simulink model "Assign_Task3and4"  (R2024a)
settings: Solver=ode1  StartTime=0.0  StopTime=simTime  FixedStep=Ts  MaxStep=Ts  RelTol=1e-3
model workspace (MAT data in the model file):
  wsw = 2000
values from neighbouring files (symbols this model uses):
  fg = 50    [Parameters.m]
  generator_inertia = 5    [Parameters.m]
  kd = 0    [Parameters.m]
  ki = 0    [Parameters.m]
  kp = 1/R    (= 20)    [Parameters.m]
  R = 0.05    [Parameters.m]
  S0non = 1000e6    (= 1000000000)    [Parameters.m]
  simTime = 60    [Parameters.m]
  Ts = 20e-6    (= 2e-05)    [Parameters.m]
  Vhv = 22e3    (= 22000)    [Parameters.m]
  Vmv = 22e3    (= 22000)    [Parameters.m]
libraries: simulink_extras x8, spsCurrentMeasurementLib x6, spsGroundLib x6, spsVoltageMeasurementLib x6, spsThreePhaseParallelRLCLoadLib x6, simulink x3, spsPower3phInstantaneousLib x2, spsSynchronousMachinepuStandardLib x2, spsThreePhaseBreakerLib x2, spsThreePhaseDynamicLoadLib x1, slpidlib x1, eeGeneralControl x1
settings Model: Creator=Vinicius  LastModifiedBy=citcea
settings SolverCC: AlgebraicLoopSolver=TrustRegion
settings DataIOCC: InitialState=out_EMTsteady50VSC.xFinal  SaveOperatingPoint=on  SaveOutput=off  SignalLogging=off  DSMLogging=off  TimeSaveName=t
settings OptimizationCC: BlockReduction=off
settings ModelReferenceCC: EnableRefExpFcnMdlSchedulingChecks=on
settings RTWCC: BuildConfiguration=Faster Runs  GPUComputeCapability=3.5  DLArmComputeVersion=19.05

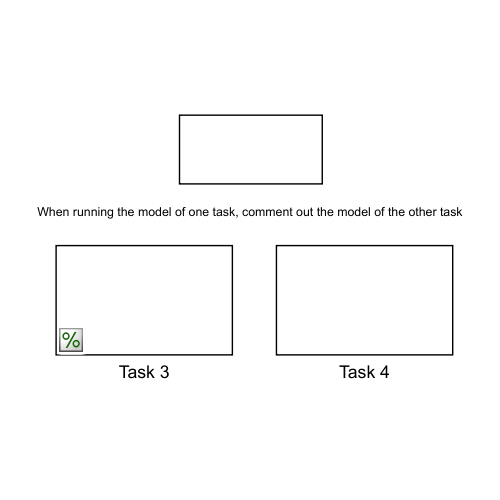
[thumbnail: Simulink's stored preview of the top-level diagram]
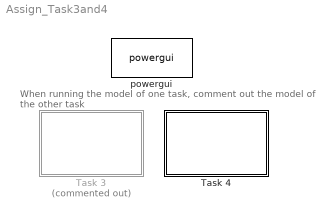
== system Assign_Task3and4 ==
  note: When running the model of one task, comment out the model of the other task
  Task 3 : Subsystem  Commented=on
  Task 4 : Subsystem
  powergui : sps_lib/powergui  Priority=1  SimulationMode=Discrete  SampleTime=Ts  frequency=60  Iterations=50  frequencyindice=50  Pbase=100e6  ErrMax=0.0001  UnitsV=kV  UnitsW=MW  buscounter=0  FunctionMessages=off  echomessages=off  EnableUseOfTLC=off  CurrentSourceSwitches=off  DisableSnubberDevices=off  DisableRonSwitches=off  DisableVfSwitches=off  DisplayEquations=off  AutomaticDiscreteSolvers=off  SolverType=Tustin/Backward Euler (TBE)  Interpol=off  ExternalGateDelay=off  methode=off  Ts=100  x0status=blocks  SPID=on  SwTol=0  HookPort=off  NonlinearTolerance=1e-4  nMaxIteration=100  ContinueOnMaxIteration=off  RestoreLinks=warning  ResistiveCurrentMeasurement=off  Frange=[0:2:500]  Ylog=off  Xlog=on  ShowGrid=off  save=off  variable=ZData  structure=0  ZoomFFT=off  StartTime=0.0  cycles=1  DisplayStyle=1  fundamental=60  FreqAxis=off  MaxFrequency=1000  frequencyindicesteady=1  RmsSteady=1  display=off

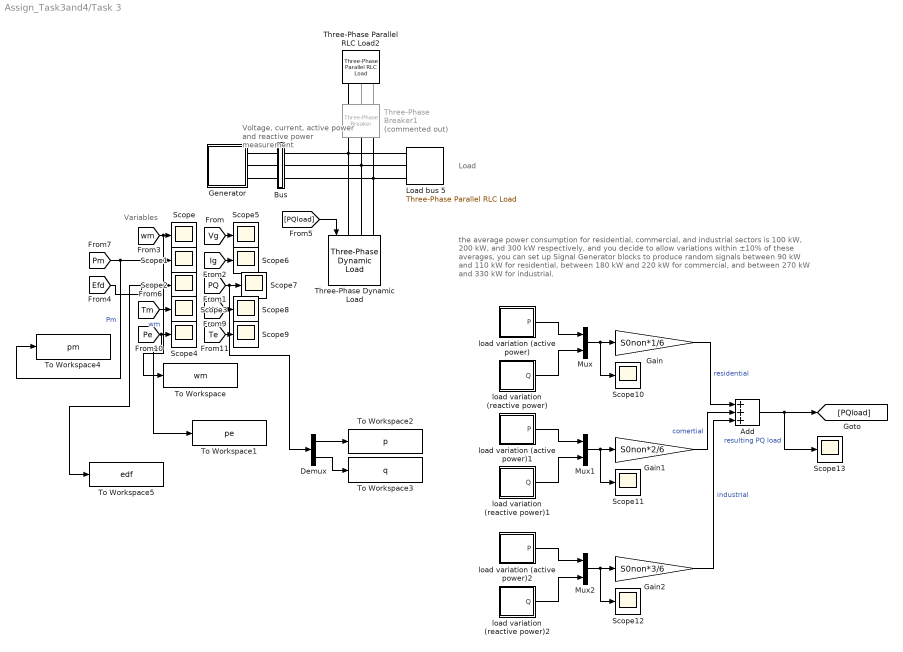
== system Assign_Task3and4/Task 3 ==
  note: the average power consumption for residential, commercial, and industrial sectors is 100 kW, 200 kW, and 300 kW respectively, and you decide to allow variations within ±10% of these averages, you can set up Signal Generator blocks to produce random signals between 90 kW and 110 kW for residential, between 180 kW and 220 kW for commercial, and between 270 kW and 330 kW for industrial.
  note: Variables
  note: Voltage, current, active power and reactive power measurement
  note: Load
  Add : Sum  Inputs=+++
  Bus : Subsystem
  Demux : Demux  Outputs=2
  Gain : Gain  Gain=S0non*1/6
  Gain1 : Gain  Gain=S0non*2/6
  Gain2 : Gain  Gain=S0non*3/6
  Generator : Subsystem
      mask Display: disp('SG')
  Load bus 5 : spsThreePhaseParallelRLCLoadLib/Three-Phase Parallel RLC Load  LConnTagsString=A|B|C  Configuration=Y (grounded)  NominalVoltage=Vmv  Vabc=[1e3 1e3 1e3]  Vabcp=[1e3 1e3 1e3]  NominalFrequency=fg  UnbalancedPower=off  ActivePower=300e6  InductivePower=50e6  CapacitivePower=0  Pabc=[10e3 9e3 11e3]  QLabc=[100 90 110]  QCabc=[100 90 110]  Pabcp=[10e3 9e3 11e3]  QLabcp=[100 90 110]  QCabcp=[100 90 110]  Measurements=None  LoadType=constant PQ
  Mux : Mux  Inputs=2
  Mux1 : Mux  Inputs=2
  Mux2 : Mux  Inputs=2
  Scope{,1..13} (14 alike) : Scope
  Three-Phase Dynamic Load : spsThreePhaseDynamicLoadLib/Three-Phase Dynamic Load  NominalVoltage=[Vmv 50 ]  ActiveReactivePowers=[0.3 0.01]*S0non  PositiveSequence=[1.0 0]  ExternalControl=on  NpNq=[1.3 2]  TimeConstants="[0  0  0  0]"  MinimumVoltage=0.7  Tfilter=1e-4  LoadFlowParameters=[4,0,0,0,0]
      settings: LibrarySourceBlock=|
      | sps_lib/Passives/Three-Phase
      | Dynamic Load
  Three-Phase Parallel RLC Load2 : spsThreePhaseParallelRLCLoadLib/Three-Phase Parallel RLC Load  LConnTagsString=A|B|C  Configuration=Y (grounded)  NominalVoltage=Vmv  Vabc=[1 1 1]*Vhv  Vabcp=[1e3 1e3 1e3]  NominalFrequency=fg  UnbalancedPower=off  ActivePower=first_load_active_power  InductivePower=0  CapacitivePower=0  Pabc=[10 10 10]*1e6  QLabc=[1 1 1]*1e6  QCabc=[0 0 0]  Pabcp=[10e3 9e3 11e3]  QLabcp=[100 90 110]  QCabcp=[100 90 110]  Measurements=None  LoadType=constant Z
  Three-Phase Breaker1 : spsThreePhaseBreakerLib/Three-Phase Breaker  Commented=on  InitialState=open  SwitchA=on  SwitchB=on  SwitchC=on  SwitchTimes=simTime/2  External=off  BreakerResistance=0.001  SnubberResistance=1e7  SnubberCapacitance=inf  Measurements=None
  To Workspace : ToWorkspace  VariableName=wm  SaveFormat=Timeseries  SampleTime=-1
  To Workspace1 : ToWorkspace  VariableName=pe  SaveFormat=Timeseries  SampleTime=-1
  To Workspace2 : ToWorkspace  VariableName=p  SaveFormat=Timeseries  SampleTime=-1
  To Workspace3 : ToWorkspace  VariableName=q  SaveFormat=Timeseries  SampleTime=-1
  To Workspace4 : ToWorkspace  VariableName=pm  SaveFormat=Timeseries  SampleTime=-1
  To Workspace5 : ToWorkspace  VariableName=edf  SaveFormat=Timeseries  SampleTime=-1
  load variation (active power) : Subsystem
  load variation (active power)1 : Subsystem
  load variation (active power)2 : Subsystem
  load variation (reactive power) : Subsystem
  load variation (reactive power)1 : Subsystem
  load variation (reactive power)2 : Subsystem
  wires:
  Mux/1 -> Scope10/1, Gain/1
  load variation (reactive power)/1(Q) -> Mux/2
  load variation (active power)/1(P) -> Mux/1
  [PQload] -> Three-Phase Dynamic Load/1
  [wm] -> To Workspace/1, Scope/1  "wm"
  [Pm] -> To Workspace4/1, Scope1/1  "Pm"
  [Tm] -> Scope3/1
  [Pe] -> To Workspace1/1, Scope4/1
  [Vg] -> Scope5/1
  [Ig] -> Scope6/1
  [Ifd] -> Scope8/1
  [Te] -> Scope9/1
  Demux/1 -> To Workspace2/1
  [PQ] -> Demux/1, Scope7/1
  Demux/2 -> To Workspace3/1
  Mux1/1 -> Gain1/1, Scope11/1
  load variation (active power)1/1(P) -> Mux1/1
  Gain1/1 -> Add/2  "comertial"
  load variation (reactive power)1/1(Q) -> Mux1/2
  Add/1 -> Scope13/1, [PQload]  "resulting PQ load"
  Gain/1 -> Add/1  "residential"
  Gain2/1 -> Add/3  "industrial"
  Mux2/1 -> Gain2/1, Scope12/1
  load variation (active power)2/1(P) -> Mux2/1
  load variation (reactive power)2/1(Q) -> Mux2/2
  [Efd] -> Scope2/1, To Workspace5/1
  connections:
  Load bus 5/LConn1 -- Bus/RConn1 -- Three-Phase Dynamic Load/LConn1 -- Three-Phase Breaker1/LConn1
  Load bus 5/LConn2 -- Bus/RConn2 -- Three-Phase Dynamic Load/LConn2 -- Three-Phase Breaker1/LConn2
  Generator/RConn1 -- Bus/LConn1
  Load bus 5/LConn3 -- Bus/RConn3 -- Three-Phase Dynamic Load/LConn3 -- Three-Phase Breaker1/LConn3
  Generator/RConn2 -- Bus/LConn2
  Generator/RConn3 -- Bus/LConn3
  Three-Phase Breaker1/RConn2 -- Three-Phase Parallel RLC Load2/LConn2
  Three-Phase Breaker1/RConn3 -- Three-Phase Parallel RLC Load2/LConn3
  Three-Phase Parallel RLC Load2/LConn1 -- Three-Phase Breaker1/RConn1

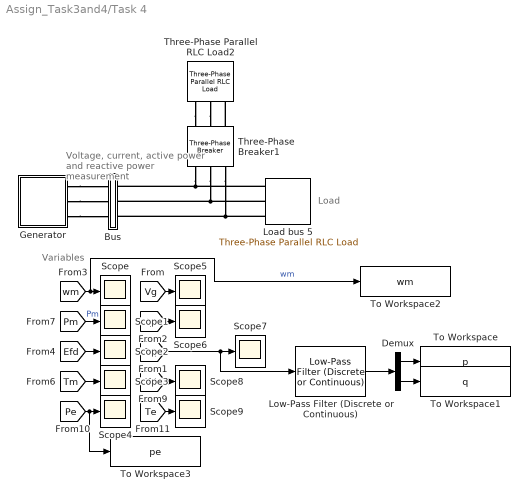
== system Assign_Task3and4/Task 4 ==
  note: Variables
  note: Voltage, current, active power and reactive power measurement
  note: Load
  Bus : Subsystem
  Demux : Demux  Outputs=2
  Generator : Subsystem
      mask Display: disp('SG')
  Load bus 5 : spsThreePhaseParallelRLCLoadLib/Three-Phase Parallel RLC Load  LConnTagsString=A|B|C  Configuration=Y (grounded)  NominalVoltage=Vmv  Vabc=[1e3 1e3 1e3]  Vabcp=[1e3 1e3 1e3]  NominalFrequency=fg  UnbalancedPower=off  ActivePower=S0non*0.5  InductivePower=0  CapacitivePower=0  Pabc=[10e3 9e3 11e3]  QLabc=[100 90 110]  QCabc=[100 90 110]  Pabcp=[10e3 9e3 11e3]  QLabcp=[100 90 110]  QCabcp=[100 90 110]  Measurements=None  LoadType=constant PQ
  Low-Pass Filter (Discrete or Continuous) : eeGeneralControl/Low-Pass Filter (Discrete or Continuous)  K=1  T=1  B=inf  A=-inf  init_option=Inherited from block input  x0=0  Ts=-1
  Scope{,1..9} (10 alike) : Scope
  Three-Phase Parallel RLC Load2 : spsThreePhaseParallelRLCLoadLib/Three-Phase Parallel RLC Load  LConnTagsString=A|B|C  Configuration=Y (grounded)  NominalVoltage=Vmv  Vabc=[1 1 1]*Vhv  Vabcp=[1e3 1e3 1e3]  NominalFrequency=fg  UnbalancedPower=off  ActivePower=(S0non*0.2)*0.8  InductivePower=(S0non*0.2)*(1-0.8)  CapacitivePower=0  Pabc=[10 10 10]*1e6  QLabc=[1 1 1]*1e6  QCabc=[0 0 0]  Pabcp=[10e3 9e3 11e3]  QLabcp=[100 90 110]  QCabcp=[100 90 110]  Measurements=None  LoadType=constant Z
  Three-Phase Breaker1 : spsThreePhaseBreakerLib/Three-Phase Breaker  InitialState=open  SwitchA=on  SwitchB=on  SwitchC=on  SwitchTimes=simTime/2  External=off  BreakerResistance=0.001  SnubberResistance=1e7  SnubberCapacitance=inf  Measurements=None
  To Workspace : ToWorkspace  VariableName=p  SaveFormat=Timeseries  SampleTime=-1
  To Workspace1 : ToWorkspace  VariableName=q  SaveFormat=Timeseries  SampleTime=-1
  To Workspace2 : ToWorkspace  VariableName=wm  SaveFormat=Timeseries  SampleTime=-1
  To Workspace3 : ToWorkspace  VariableName=pe  SaveFormat=Timeseries  SampleTime=-1
  wires:
  [wm] -> To Workspace2/1, Scope/1  "wm"
  [Pm] -> Scope1/1  "Pm"
  [Efd] -> Scope2/1
  [Tm] -> Scope3/1
  [Pe] -> To Workspace3/1, Scope4/1
  [Vg] -> Scope5/1
  [Ig] -> Scope6/1
  [PQ] -> Low-Pass Filter (Discrete or Continuous)/1, Scope7/1
  [Ifd] -> Scope8/1
  [Te] -> Scope9/1
  Demux/1 -> To Workspace/1
  Demux/2 -> To Workspace1/1
  Low-Pass Filter (Discrete or Continuous)/1 -> Demux/1
  connections:
  Generator/RConn1 -- Bus/LConn1
  Generator/RConn2 -- Bus/LConn2
  Generator/RConn3 -- Bus/LConn3
  Load bus 5/LConn1 -- Bus/RConn1 -- Three-Phase Breaker1/LConn1
  Load bus 5/LConn2 -- Three-Phase Breaker1/LConn2 -- Bus/RConn2
  Load bus 5/LConn3 -- Three-Phase Breaker1/LConn3 -- Bus/RConn3
  Three-Phase Breaker1/RConn3 -- Three-Phase Parallel RLC Load2/LConn3
  Three-Phase Parallel RLC Load2/LConn1 -- Three-Phase Breaker1/RConn1
  Three-Phase Parallel RLC Load2/LConn2 -- Three-Phase Breaker1/RConn2

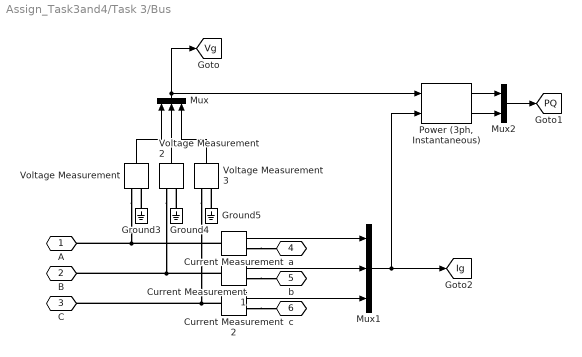
== system Assign_Task3and4/Task 3/Bus ==
  Current Measurement : spsCurrentMeasurementLib/Current Measurement  PhasorSimulation=off  OutputType=Complex  PSBequivalent=0
  Current Measurement1 : spsCurrentMeasurementLib/Current Measurement  PhasorSimulation=off  OutputType=Complex  PSBequivalent=0
  Current Measurement2 : spsCurrentMeasurementLib/Current Measurement  PhasorSimulation=off  OutputType=Complex  PSBequivalent=0
  Ground3 : spsGroundLib/Ground  LConnTagsString=a
  Ground4 : spsGroundLib/Ground  LConnTagsString=a
  Ground5 : spsGroundLib/Ground  LConnTagsString=a
  Mux : Mux  Inputs=3
  Mux1 : Mux  Inputs=3
  Mux2 : Mux  Inputs=2
  "Power (3ph, Instantaneous)" : spsPower3phInstantaneousLib/Power (3ph, Instantaneous)
  Voltage Measurement : spsVoltageMeasurementLib/Voltage Measurement  PhasorSimulation=off  OutputType=Complex  PSBequivalent=0
  Voltage Measurement2 : spsVoltageMeasurementLib/Voltage Measurement  PhasorSimulation=off  OutputType=Complex  PSBequivalent=0
  Voltage Measurement3 : spsVoltageMeasurementLib/Voltage Measurement  PhasorSimulation=off  OutputType=Complex  PSBequivalent=0
  A : PMIOPort  Side=Left
  B : PMIOPort  Port=2  Side=Left
  C : PMIOPort  Port=3  Side=Left
  a : PMIOPort  Port=4  Side=Right
  b : PMIOPort  Port=5  Side=Right
  c : PMIOPort  Port=6  Side=Right
  tag scope: Ig=global, PQ=global, Vg=global
  wires:
  Voltage Measurement3/1 -> Mux/3
  Voltage Measurement2/1 -> Mux/2
  Voltage Measurement/1 -> Mux/1
  Mux/1 -> [Vg], "Power (3ph, Instantaneous)"/1
  Current Measurement/1 -> Mux1/1
  Current Measurement1/1 -> Mux1/2
  Current Measurement2/1 -> Mux1/3
  Mux1/1 -> [Ig], "Power (3ph, Instantaneous)"/2
  "Power (3ph, Instantaneous)"/1 -> Mux2/1
  "Power (3ph, Instantaneous)"/2 -> Mux2/2
  Mux2/1 -> [PQ]
  connections:
  Ground5/LConn1 -- Voltage Measurement3/LConn2
  Current Measurement/RConn1 -- a/RConn1
  Voltage Measurement2/LConn1 -- Current Measurement1/LConn1 -- B/RConn1
  Voltage Measurement3/LConn1 -- Current Measurement2/LConn1 -- C/RConn1
  Voltage Measurement/LConn1 -- Current Measurement/LConn1 -- A/RConn1
  Ground3/LConn1 -- Voltage Measurement/LConn2
  Ground4/LConn1 -- Voltage Measurement2/LConn2
  Current Measurement1/RConn1 -- b/RConn1
  Current Measurement2/RConn1 -- c/RConn1

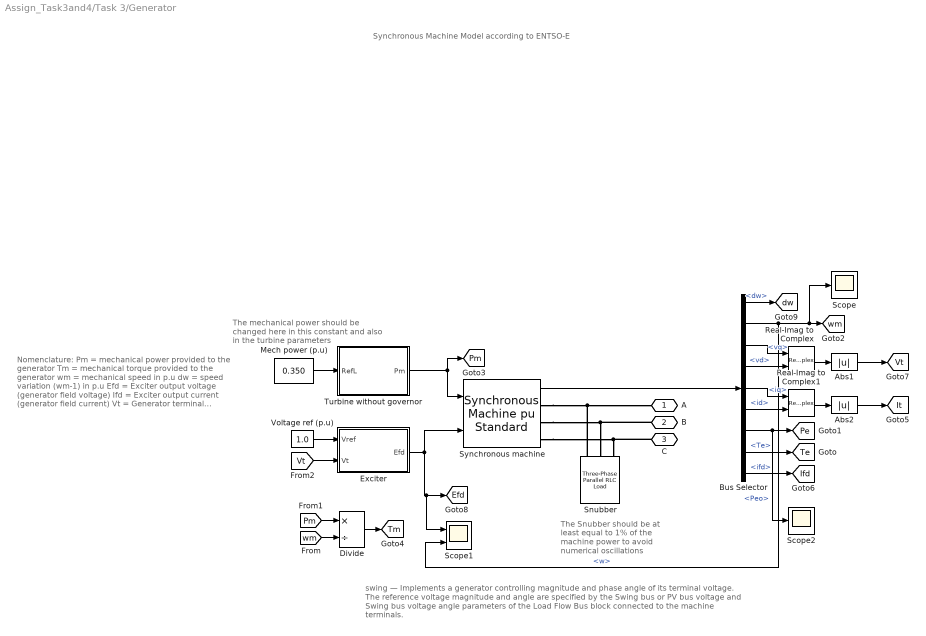
== system Assign_Task3and4/Task 3/Generator ==
  note: swing — Implements a generator controlling magnitude and phase angle of its terminal voltage. The reference voltage magnitude and angle are specified by the Swing bus or PV bus voltage and Swing bus voltage angle parameters of the Load Flow Bus block connected to the machine terminals.
  note: The Snubber should be at least equal to 1% of the machine power to avoid numerical oscillations
  note: Nomenclature:
      |
      | Pm = mechanical power provided to the generator
      | Tm = mechanical torque provided to the generator
      | wm = mechanical speed in p.u
      | dw = speed variation (wm-1) in p.u
      | Efd = Exciter output voltage (generator field voltage)
      | Ifd = Exciter output current (generator field current)
      | Vt = Generator terminal voltage
      | It = Generator terminal current
      | Vref = Voltage regulator reference signal
  note: Synchronous Machine Model according to ENTSO-E
  note: The mechanical power should be changed here in this constant and also in the turbine parameters
  Abs1 : Abs  SaturateOnIntegerOverflow=off
  Abs2 : Abs  SaturateOnIntegerOverflow=off
  Bus Selector : BusSelector  OutputSignals=dw,w,vq,vd,iq,id,Peo,Te,ifd
  Divide : Product  Inputs=*/
  Exciter : Subsystem  mask{K=200, Ta=3, Tb=10, Te=0.05, Emin=-4, Emax=4, Vf0=1.30534}
      mask prompts: K "Controller gain (K)"; Ta "Filter derivative time constant (Ta)(sec)"; Tb "Filter delay time (Tb)(sec)"; Te "Exciter time constant (Te)(sec)"; Emin "Controller minimum output (Emin)"; Emax "Controller maximum output (Emax)"; Vf0 "Initial output (p.u)"
      mask Display:
      | disp('AVR')
      | 
      | port_label('input',1,'Vref')
      | port_label('input',2,'Vc')
      | 
      | port_label('output',1,'Efd')
  Mech power (p.u) : Constant  Value=0.350  VectorParams1D=off
  Real-Imag to Complex : RealImagToComplex
  Real-Imag to Complex1 : RealImagToComplex
  Scope : Scope
  Scope1 : Scope  NumInputPorts=2
  Scope2 : Scope
  Snubber : spsThreePhaseParallelRLCLoadLib/Three-Phase Parallel RLC Load  LConnTagsString=A|B|C  Configuration=Y (grounded)  NominalVoltage=Vmv  Vabc=[1 1 1]*Vmv  Vabcp=[1e3 1e3 1e3]  NominalFrequency=fg  UnbalancedPower=off  ActivePower=0.05*S0non  InductivePower=0  CapacitivePower=0  Pabc=[10e3 10e3 10e3]  QLabc=[0 0 0]  QCabc=[0 0 0]  Pabcp=[10e3 9e3 11e3]  QLabcp=[100 90 110]  QCabcp=[100 90 110]  Measurements=None  LoadType=constant Z
  Synchronous machine : spsSynchronousMachinepuStandardLib/Synchronous Machine pu Standard  PresetModel=No  MechanicalLoad=Mechanical power Pm  ShowDetailedParameters=on  RotorType=Salient-pole  Units=per unit standard parameters  MeasurementBus=on  NominalParameters=[S0non Vmv fg]  Reactances1=[ 1.81, 0.3, 0.23, 1.76, 0.65, 0.25, 0.15 ]  Reactances2=[2.0 0.35 0.25 1.8 0.3 0.15]  dAxisTimeConstants=Short-circuit  qAxisTimeConstants=Short-circuit  TimeConstants1="[ 4.4849  0.0681  0.1  ]"  TimeConstants2=[ 8.0, 0.03, 1.0, 0.07 ]  TimeConstants3="[  4.49  0.0681  0.0513  ]"  TimeConstants4=[ 8.0, 0.03, 0.3371, 0.0295 ]  TimeConstants5=[ 1.01, 0.053, 0.1 ]  TimeConstants6=[ 1.3201, 0.023, 1.0, 0.07 ]  TimeConstants7=[0.9 0.03 0.05]  TimeConstants8=[ 1.3201, 0.0231, 0.3371, 0.0295 ]  StatorResistance=0.01  Mechanical=[generator_inertia 0 2]  PolePairs=20  InitialConditions=[0 -60.0721 0.353553 0.353553 0.353553 -8.1301 -128.13 111.87 1.30534]  SetSaturation=off  Saturation=[0.6404,0.7127,0.8441,0.9214,0.9956,1.082,1.19,1.316,1.457;0.7,0.7698,0.8872,0.9466,0.9969,1.046,1.1,1.151,1.201]  LoadFlowParameters=[2 47500000 0 0 0]  TsPowergui=0  TsBlock=-1  IterativeModel=Trapezoidal non iterative  IterativeDiscreteModel=Trapezoidal non iterative  BusType=swing  Pref=475e6  Qref=0  Qmin=-inf  Qmax=inf  PLF=0  QLF=0
  Turbine without governor : Subsystem  mask{R=0.05, T1=0.5, T2=3, T3=10, Dt=0, Vmin=0, Vmax=10, P0=0.351}
      mask prompts: R "Controller droop (R)"; T1 "Governor time constant (T1)(sec)"; T2 "Turbine derivative time constant (T2)(sec)"; T3 "Turbine delay time constant (T3)(sec)"; Dt "Frictional losses factor (Dt)"; Vmin "Minimum gate limit (Vmin)(p.u)"; Vmax "Maximum gate limit (Vmax)(p.u)"; P0 "Initial power (p.u)"
      mask Display:
      | disp('Turbine')
      | 
      | port_label('input',1,'Pref')
      | 
      | port_label('output',1,'Pm')
  Voltage ref (p.u) : Constant  Value=1.0
  A : PMIOPort  Side=Right
  B : PMIOPort  Port=2  Side=Right
  C : PMIOPort  Port=3  Side=Right
  tag scope: Efd=global, Ifd=global, It=global, Pe=global, Pm=global, Te=global, Tm=global, Vt=global, dw=global, wm=global
  wires:
  Exciter/1(Efd) -> Synchronous machine/2, Scope1/1, [Efd]
  Voltage ref (p.u)/1 -> Exciter/1(Vref)
  Turbine without governor/1(Pm) -> Synchronous machine/1, [Pm]
  Mech power (p.u)/1 -> Turbine without governor/1(RefL)
  [Pm] -> Divide/1
  [wm] -> Divide/2
  Divide/1 -> [Tm]
  Bus Selector/4 -> Real-Imag to Complex/2  "<vd>"
  Abs2/1 -> [It]
  Real-Imag to Complex1/1 -> Abs2/1
  Real-Imag to Complex/1 -> Abs1/1
  Bus Selector/6 -> Real-Imag to Complex1/2  "<id>"
  Bus Selector/2 -> Scope/1, [wm], Scope1/2  "<w>"
  Bus Selector/8 -> [Te]  "<Te>"
  Bus Selector/3 -> Real-Imag to Complex/1  "<vq>"
  Bus Selector/7 -> Scope2/1, [Pe]  "<Peo>"
  Bus Selector/5 -> Real-Imag to Complex1/1  "<iq>"
  Synchronous machine/1 -> Bus Selector/1
  Bus Selector/9 -> [Ifd]  "<ifd>"
  Abs1/1 -> [Vt]
  [Vt] -> Exciter/2(Vt)
  Bus Selector/1 -> [dw]  "<dw>"
  connections:
  B/RConn1 -- Synchronous machine/RConn2 -- Snubber/LConn2
  C/RConn1 -- Synchronous machine/RConn3 -- Snubber/LConn3
  Snubber/LConn1 -- Synchronous machine/RConn1 -- A/RConn1

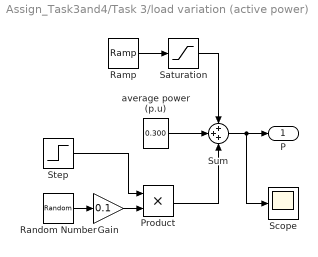
== system Assign_Task3and4/Task 3/load variation (active power) ==
  Gain : Gain  Gain=0.1
  Product : Product
  Ramp : simulink/Sources/Ramp  slope=0.005  start=5  InitialOutput=0
  Random Number : RandomNumber  Variance=0.2  SampleTime=0.01
  Saturation : Saturate  UpperLimit=0.1  LowerLimit=0
  Scope : Scope
  Step : Step  Time=simTime/4  SampleTime=0
  Sum : Sum  Inputs=+++
  average power (p.u) : Constant  Value=0.300  VectorParams1D=off
  P : Outport
  wires:
  Step/1 -> Product/1
  Gain/1 -> Product/2
  Random Number/1 -> Gain/1
  Sum/1 -> Scope/1, P/1
  average power (p.u)/1 -> Sum/2
  Product/1 -> Sum/3
  Ramp/1 -> Saturation/1
  Saturation/1 -> Sum/1

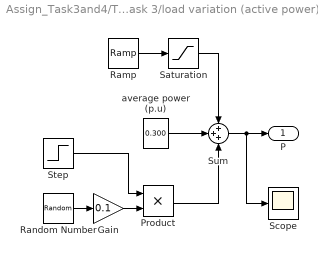
== system Assign_Task3and4/Task 3/load variation (active power)1 ==
  Gain : Gain  Gain=0.1
  Product : Product
  Ramp : simulink/Sources/Ramp  slope=0.005  start=5  InitialOutput=0
  Random Number : RandomNumber  Variance=0.5  SampleTime=0.05
  Saturation : Saturate  UpperLimit=0.1  LowerLimit=0
  Scope : Scope
  Step : Step  Time=simTime/4  SampleTime=0
  Sum : Sum  Inputs=+++
  average power (p.u) : Constant  Value=0.300  VectorParams1D=off
  P : Outport
  wires:
  Step/1 -> Product/1
  Gain/1 -> Product/2
  Random Number/1 -> Gain/1
  Sum/1 -> Scope/1, P/1
  average power (p.u)/1 -> Sum/2
  Product/1 -> Sum/3
  Ramp/1 -> Saturation/1
  Saturation/1 -> Sum/1

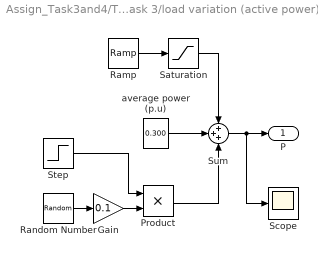
== system Assign_Task3and4/Task 3/load variation (active power)2 ==
  Gain : Gain  Gain=0.1
  Product : Product
  Ramp : simulink/Sources/Ramp  slope=0.005  start=5  InitialOutput=0
  Random Number : RandomNumber  Variance=0.4  SampleTime=0.1
  Saturation : Saturate  UpperLimit=0.1  LowerLimit=0
  Scope : Scope
  Step : Step  Time=simTime/4  SampleTime=0
  Sum : Sum  Inputs=+++
  average power (p.u) : Constant  Value=0.300  VectorParams1D=off
  P : Outport
  wires:
  Step/1 -> Product/1
  Gain/1 -> Product/2
  Random Number/1 -> Gain/1
  Sum/1 -> Scope/1, P/1
  average power (p.u)/1 -> Sum/2
  Product/1 -> Sum/3
  Ramp/1 -> Saturation/1
  Saturation/1 -> Sum/1

== system Assign_Task3and4/Task 3/load variation (reactive power) ==
  Gain : Gain  Gain=0.1
  Product : Product
  Random Number : RandomNumber  Variance=0.2  SampleTime=0.01
  Step : Step  Time=simTime/4  SampleTime=0
  Sum : Sum  Inputs=|++
  average power (p.u) : Constant  Value=0.05  VectorParams1D=off
  Q : Outport
  wires:
  Step/1 -> Product/1
  Gain/1 -> Product/2
  Random Number/1 -> Gain/1
  average power (p.u)/1 -> Sum/1
  Product/1 -> Sum/2
  Sum/1 -> Q/1

== system Assign_Task3and4/Task 3/load variation (reactive power)1 ==
  Gain : Gain  Gain=0.1
  Product : Product
  Random Number : RandomNumber  Variance=0.5  SampleTime=0.05
  Step : Step  Time=simTime/4  SampleTime=0
  Sum : Sum  Inputs=|++
  average power (p.u) : Constant  Value=0.05  VectorParams1D=off
  Q : Outport
  wires:
  Step/1 -> Product/1
  Gain/1 -> Product/2
  Random Number/1 -> Gain/1
  average power (p.u)/1 -> Sum/1
  Product/1 -> Sum/2
  Sum/1 -> Q/1

== system Assign_Task3and4/Task 3/load variation (reactive power)2 ==
  Gain : Gain  Gain=0.1
  Product : Product
  Random Number : RandomNumber  Variance=0.4  SampleTime=0.1
  Step : Step  Time=simTime/4  SampleTime=0
  Sum : Sum  Inputs=|++
  average power (p.u) : Constant  Value=0.05  VectorParams1D=off
  Q : Outport
  wires:
  Step/1 -> Product/1
  Gain/1 -> Product/2
  Random Number/1 -> Gain/1
  average power (p.u)/1 -> Sum/1
  Product/1 -> Sum/2
  Sum/1 -> Q/1

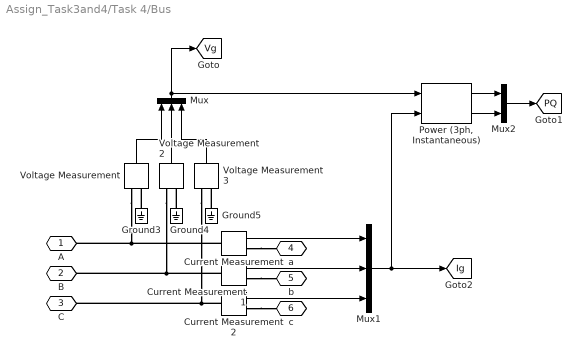
== system Assign_Task3and4/Task 4/Bus ==
  Current Measurement : spsCurrentMeasurementLib/Current Measurement  PhasorSimulation=off  OutputType=Complex  PSBequivalent=0
  Current Measurement1 : spsCurrentMeasurementLib/Current Measurement  PhasorSimulation=off  OutputType=Complex  PSBequivalent=0
  Current Measurement2 : spsCurrentMeasurementLib/Current Measurement  PhasorSimulation=off  OutputType=Complex  PSBequivalent=0
  Ground3 : spsGroundLib/Ground  LConnTagsString=a
  Ground4 : spsGroundLib/Ground  LConnTagsString=a
  Ground5 : spsGroundLib/Ground  LConnTagsString=a
  Mux : Mux  Inputs=3
  Mux1 : Mux  Inputs=3
  Mux2 : Mux  Inputs=2
  "Power (3ph, Instantaneous)" : spsPower3phInstantaneousLib/Power (3ph, Instantaneous)
  Voltage Measurement : spsVoltageMeasurementLib/Voltage Measurement  PhasorSimulation=off  OutputType=Complex  PSBequivalent=0
  Voltage Measurement2 : spsVoltageMeasurementLib/Voltage Measurement  PhasorSimulation=off  OutputType=Complex  PSBequivalent=0
  Voltage Measurement3 : spsVoltageMeasurementLib/Voltage Measurement  PhasorSimulation=off  OutputType=Complex  PSBequivalent=0
  A : PMIOPort  Side=Left
  B : PMIOPort  Port=2  Side=Left
  C : PMIOPort  Port=3  Side=Left
  a : PMIOPort  Port=4  Side=Right
  b : PMIOPort  Port=5  Side=Right
  c : PMIOPort  Port=6  Side=Right
  tag scope: Ig=global, PQ=global, Vg=global
  wires:
  Voltage Measurement3/1 -> Mux/3
  Voltage Measurement2/1 -> Mux/2
  Voltage Measurement/1 -> Mux/1
  Mux/1 -> [Vg], "Power (3ph, Instantaneous)"/1
  Current Measurement/1 -> Mux1/1
  Current Measurement1/1 -> Mux1/2
  Current Measurement2/1 -> Mux1/3
  Mux1/1 -> [Ig], "Power (3ph, Instantaneous)"/2
  "Power (3ph, Instantaneous)"/1 -> Mux2/1
  "Power (3ph, Instantaneous)"/2 -> Mux2/2
  Mux2/1 -> [PQ]
  connections:
  Ground5/LConn1 -- Voltage Measurement3/LConn2
  Current Measurement/RConn1 -- a/RConn1
  Voltage Measurement2/LConn1 -- Current Measurement1/LConn1 -- B/RConn1
  Voltage Measurement3/LConn1 -- Current Measurement2/LConn1 -- C/RConn1
  Voltage Measurement/LConn1 -- Current Measurement/LConn1 -- A/RConn1
  Ground3/LConn1 -- Voltage Measurement/LConn2
  Ground4/LConn1 -- Voltage Measurement2/LConn2
  Current Measurement1/RConn1 -- b/RConn1
  Current Measurement2/RConn1 -- c/RConn1

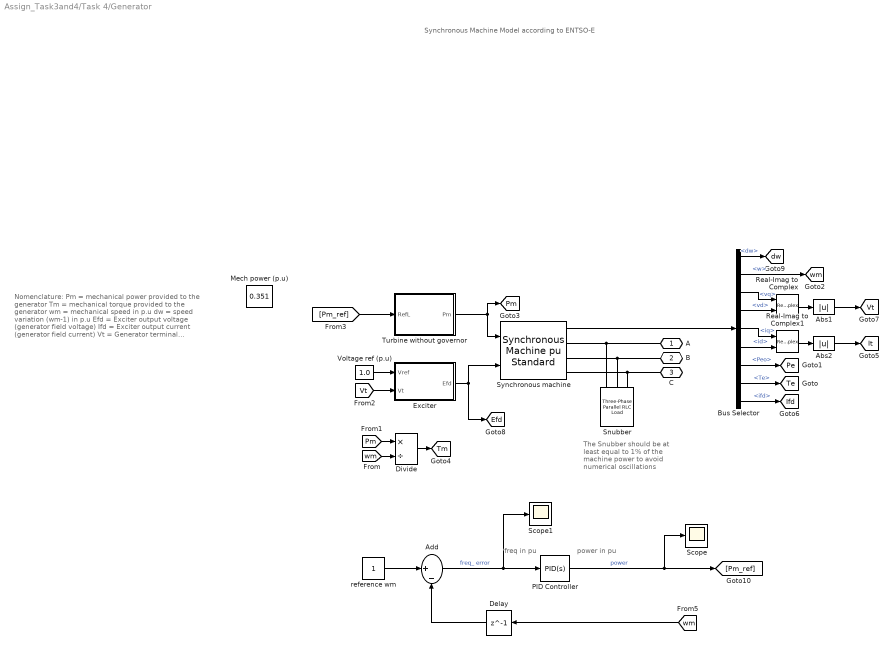
== system Assign_Task3and4/Task 4/Generator ==
  note: freq in pu
  note: power in pu
  note: The Snubber should be at least equal to 1% of the machine power to avoid numerical oscillations
  note: Nomenclature:
      |
      | Pm = mechanical power provided to the generator
      | Tm = mechanical torque provided to the generator
      | wm = mechanical speed in p.u
      | dw = speed variation (wm-1) in p.u
      | Efd = Exciter output voltage (generator field voltage)
      | Ifd = Exciter output current (generator field current)
      | Vt = Generator terminal voltage
      | It = Generator terminal current
      | Vref = Voltage regulator reference signal
  note: Synchronous Machine Model according to ENTSO-E
  Abs1 : Abs  SaturateOnIntegerOverflow=off
  Abs2 : Abs  SaturateOnIntegerOverflow=off
  Add : Sum  Inputs=|+-
  Bus Selector : BusSelector  OutputSignals=dw,w,vq,vd,iq,id,Peo,Te,ifd
  Delay : Delay  DelayLength=1
  Divide : Product  Inputs=*/
  Exciter : Subsystem  mask{K=200, Ta=3, Tb=10, Te=0.05, Emin=-4, Emax=4, Vf0=1.30534}
      mask prompts: K "Controller gain (K)"; Ta "Filter derivative time constant (Ta)(sec)"; Tb "Filter delay time (Tb)(sec)"; Te "Exciter time constant (Te)(sec)"; Emin "Controller minimum output (Emin)"; Emax "Controller maximum output (Emax)"; Vf0 "Initial output (p.u)"
      mask Display:
      | disp('AVR')
      | 
      | port_label('input',1,'Vref')
      | port_label('input',2,'Vc')
      | 
      | port_label('output',1,'Efd')
  Mech power (p.u) : Constant  Value=0.351  VectorParams1D=off
  PID Controller : slpidlib/PID Controller  Controller=PID  Form=Parallel  TimeDomain=Continuous-time  UseExternalTs=off  SampleTime=-1  IntegratorMethod=Forward Euler  FilterMethod=Forward Euler  ControllerParametersSource=internal  P=kp  I=ki  UseKiTs=off  D=kd  UseExternalDerivativeSource=off  N=100  UseFilter=on  TunerSelectOption=Transfer Function Based (PID Tuner App)  InitialConditionSource=internal  InitialConditionForIntegrator=0  InitialConditionForFilter=0  DifferentiatorICPrevScaledInput=0  ExternalReset=none  TrackingMode=off  Kt=1  LimitOutput=on  SatLimitsSource=internal  UpperSaturationLimit=1  LowerSaturationLimit=0  LinearizeAsGain=on  AntiWindupMode=none  Kb=1  LimitIntegrator=off  UpperIntegratorSaturationLimit=1  LowerIntegratorSaturationLimit=0  POutMin=[]  POutMax=[]  IOutMin=[]  IOutMax=[]  DOutMin=[]  DOutMax=[]  NOutMin=[]  NOutMax=[]  SumOutMin=[]  SumOutMax=[]  SaturationOutMin=[]  SaturationOutMax=[]  PParamMin=[]  PParamMax=[]  IParamMin=[]  IParamMax=[]  DParamMin=[]  DParamMax=[]  NParamMin=[]  NParamMax=[]  KbParamMin=[]  KbParamMax=[]  KtParamMin=[]  KtParamMax=[]  KbOutMin=[]  KbOutMax=[]  KtOutMin=[]  KtOutMax=[]  IntegratorOutMin=[]  IntegratorOutMax=[]  FilterOutMin=[]  FilterOutMax=[]  SumI1OutMin=[]  SumI1OutMax=[]  SumI2OutMin=[]  SumI2OutMax=[]  SumI3OutMin=[]  SumI3OutMax=[]  SumI4OutMin=[]  SumI4OutMax=[]  SumDOutMin=[]  SumDOutMax=[]  DifferentiatorOutMin=[]  DifferentiatorOutMax=[]  FilterDiffOutCoefMin=[]  FilterDiffOutCoefMax=[]  ReciprocalOutMin=[]  ReciprocalOutMax=[]  SumDenOutMin=[]  SumDenOutMax=[]  SumNumOutMin=[]  SumNumOutMax=[]  DivideOutMin=[]  DivideOutMax=[]  UdiffTsProdOutMin=[]  UdiffTsProdOutMax=[]  NTsProdOutMin=[]  NTsProdOutMax=[]  UintegralTsProdOutMin=[]  UintegralTsProdOutMax=[]  UngainTsProdOutMin=[]  UngainTsProdOutMax=[]  ClampingZeroOutDataTypeStr=Inherit: Inherit via back propagation  ClampingZeroOutMin=[]  ClampingZeroOutMax=[]  FilterDenConstantOutDataTypeStr=Inherit: Inherit via back propagation  FilterDenConstantOutMin=[]  FilterDenConstantOutMax=[]  PCopyOutDataTypeStr=Inherit: Inherit via back propagation  PCopyOutMin=[]  PCopyOutMax=[]  NCopyOutDataTypeStr=Inherit: Inherit via back propagation  NCopyOutMin=[]  NCopyOutMax=[]  IntegratorContinuousStateAttributes=''  IntegratorStateMustResolveToSignalObject=off  IntegratorRTWStateStorageClass=Auto  FilterContinuousStateAttributes=''  FilterStateMustResolveToSignalObject=off  FilterRTWStateStorageClass=Auto  ParallelPVariant=InternalParameters  IdealPVariant=Disabled  IVariant=InternalParameters  DVariant=InternalParameters  IntegratorVariant=Continuous  SatVariant=Enabled  AWVariant=Passthrough  PCopyVariant=Disabled  TRVariant=Disabled  FdbkBlocksVariant=Forward  IdealPFdbkVariant=Disabled  SatFdbkVariant=Disabled  DerivativeFilterVariant=ContFilter  NVariant=InternalParameters  NCopyVariant=Disabled  FilterICVariant=InternalICsFilter  IntegratorICVariant=InternalICs  ExternalResetVariant=Disabled  TRSumVariant=Passthrough  SumFdbkVariant=Disabled  SumVariant=Sum_PID  TsampFilterVariant=InternalTs  TsampNgainVariant=Passthrough  TsampIntegralVariant=Disabled_SignalSpec  ExternalSaturationOutDataTypeStr=Inherit: Same as second input  DerivativeSourceVariant=ErrorSignal
  Real-Imag to Complex : RealImagToComplex
  Real-Imag to Complex1 : RealImagToComplex
  Scope : Scope
  Scope1 : Scope
  Snubber : spsThreePhaseParallelRLCLoadLib/Three-Phase Parallel RLC Load  LConnTagsString=A|B|C  Configuration=Y (grounded)  NominalVoltage=Vmv  Vabc=[1 1 1]*Vmv  Vabcp=[1e3 1e3 1e3]  NominalFrequency=fg  UnbalancedPower=off  ActivePower=0.05*S0non  InductivePower=0  CapacitivePower=0  Pabc=[10e3 10e3 10e3]  QLabc=[0 0 0]  QCabc=[0 0 0]  Pabcp=[10e3 9e3 11e3]  QLabcp=[100 90 110]  QCabcp=[100 90 110]  Measurements=None  LoadType=constant Z
  Synchronous machine : spsSynchronousMachinepuStandardLib/Synchronous Machine pu Standard  PresetModel=No  MechanicalLoad=Mechanical power Pm  ShowDetailedParameters=on  RotorType=Salient-pole  Units=per unit standard parameters  MeasurementBus=on  NominalParameters=[S0non Vmv fg]  Reactances1=[ 1.81, 0.3, 0.23, 1.76, 0.65, 0.25, 0.15 ]  Reactances2=[2.0 0.35 0.25 1.8 0.3 0.15]  dAxisTimeConstants=Short-circuit  qAxisTimeConstants=Short-circuit  TimeConstants1="[ 4.4849  0.0681  0.1  ]"  TimeConstants2=[ 8.0, 0.03, 1.0, 0.07 ]  TimeConstants3="[  4.49  0.0681  0.0513  ]"  TimeConstants4=[ 8.0, 0.03, 0.3371, 0.0295 ]  TimeConstants5=[ 1.01, 0.053, 0.1 ]  TimeConstants6=[ 1.3201, 0.023, 1.0, 0.07 ]  TimeConstants7=[0.9 0.03 0.05]  TimeConstants8=[ 1.3201, 0.0231, 0.3371, 0.0295 ]  StatorResistance=0.01  Mechanical=[generator_inertia 0 2]  PolePairs=20  InitialConditions=[0 -60.0721 0.353553 0.353553 0.353553 -8.1301 -128.13 111.87 1.30534]  SetSaturation=off  Saturation=[0.6404,0.7127,0.8441,0.9214,0.9956,1.082,1.19,1.316,1.457;0.7,0.7698,0.8872,0.9466,0.9969,1.046,1.1,1.151,1.201]  LoadFlowParameters=[2 47500000 0 0 0]  TsPowergui=0  TsBlock=-1  IterativeModel=Trapezoidal non iterative  IterativeDiscreteModel=Trapezoidal non iterative  BusType=swing  Pref=475e6  Qref=0  Qmin=-inf  Qmax=inf  PLF=0  QLF=0
  Turbine without governor : Subsystem  mask{R=R, T1=0.5, T2=3, T3=10, Dt=0, Vmin=0, Vmax=10, P0=0.351}
      mask prompts: R "Controller droop (R)"; T1 "Governor time constant (T1)(sec)"; T2 "Turbine derivative time constant (T2)(sec)"; T3 "Turbine delay time constant (T3)(sec)"; Dt "Frictional losses factor (Dt)"; Vmin "Minimum gate limit (Vmin)(p.u)"; Vmax "Maximum gate limit (Vmax)(p.u)"; P0 "Initial power (p.u)"
      mask Display:
      | disp('Turbine')
      | 
      | port_label('input',1,'Pref')
      | 
      | port_label('output',1,'Pm')
  Voltage ref (p.u) : Constant  Value=1.0
  reference wm : Constant
  A : PMIOPort  Side=Right
  B : PMIOPort  Port=2  Side=Right
  C : PMIOPort  Port=3  Side=Right
  tag scope: Efd=global, Ifd=global, It=global, Pe=global, Pm=global, Te=global, Tm=global, Vt=global, dw=global, wm=global
  wires:
  Exciter/1(Efd) -> Synchronous machine/2, [Efd]
  Voltage ref (p.u)/1 -> Exciter/1(Vref)
  Turbine without governor/1(Pm) -> Synchronous machine/1, [Pm]
  [Pm] -> Divide/1
  [wm] -> Divide/2
  Divide/1 -> [Tm]
  Bus Selector/4 -> Real-Imag to Complex/2  "<vd>"
  Abs2/1 -> [It]
  Real-Imag to Complex1/1 -> Abs2/1
  Real-Imag to Complex/1 -> Abs1/1
  Bus Selector/6 -> Real-Imag to Complex1/2  "<id>"
  Bus Selector/2 -> [wm]  "<w>"
  Bus Selector/8 -> [Te]  "<Te>"
  Bus Selector/3 -> Real-Imag to Complex/1  "<vq>"
  Bus Selector/7 -> [Pe]  "<Peo>"
  Bus Selector/5 -> Real-Imag to Complex1/1  "<iq>"
  Synchronous machine/1 -> Bus Selector/1
  Bus Selector/9 -> [Ifd]  "<ifd>"
  Abs1/1 -> [Vt]
  [Vt] -> Exciter/2(Vt)
  Bus Selector/1 -> [dw]  "<dw>"
  [Pm_ref] -> Turbine without governor/1(RefL)
  reference wm/1 -> Add/1
  Delay/1 -> Add/2
  PID Controller/1 -> Scope/1, [Pm_ref]  "power"
  [wm] -> Delay/1
  Add/1 -> Scope1/1, PID Controller/1  "freq_ error"
  connections:
  B/RConn1 -- Synchronous machine/RConn2 -- Snubber/LConn2
  C/RConn1 -- Synchronous machine/RConn3 -- Snubber/LConn3
  Snubber/LConn1 -- Synchronous machine/RConn1 -- A/RConn1

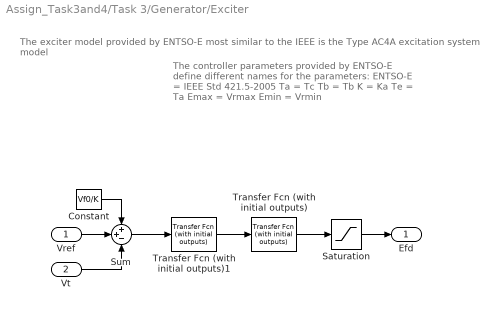
== system Assign_Task3and4/Task 3/Generator/Exciter ==
  note: The controller parameters provided by ENTSO-E
      | define different names for the parameters:
      |
      | ENTSO-E = IEEE Std 421.5-2005
      | Ta = Tc
      | Tb = Tb
      | K = Ka
      | Te = Ta
      | Emax = Vrmax
      | Emin = Vrmin
  note: The exciter model provided by ENTSO-E most similar to the IEEE is the Type AC4A excitation system model
  Vref : Inport
  Vt : Inport  Port=2
  Constant : Constant  Value=Vf0/K
  Saturation : Saturate  UpperLimit=Emax  LowerLimit=Emin
  Sum : Sum  Inputs=++-
  Transfer Fcn (with initial outputs) : simulink_extras/Additional Linear/Transfer Fcn (with initial outputs)  N=[K]  D=[Te 1]  Y0=Vf0  U0=Vf0/K
  Transfer Fcn (with initial outputs)1 : simulink_extras/Additional Linear/Transfer Fcn (with initial outputs)  N=[Ta 1]  D=[Tb 1]  Y0=Vf0/K  U0=Vf0/K
  Efd : Outport
  wires:
  Saturation/1 -> Efd/1
  Transfer Fcn (with initial outputs)1/1 -> Transfer Fcn (with initial outputs)/1
  Sum/1 -> Transfer Fcn (with initial outputs)1/1
  Transfer Fcn (with initial outputs)/1 -> Saturation/1
  Vt/1 -> Sum/3
  Vref/1 -> Sum/2
  Constant/1 -> Sum/1

== system Assign_Task3and4/Task 3/Generator/Turbine without governor ==
  note: mechanical power
  RefL : Inport
  Saturation : Saturate  UpperLimit=Vmax  LowerLimit=Vmin
  Saturation1 : Saturate  UpperLimit=1
  Transfer Fcn (with initial outputs)1 : simulink_extras/Additional Linear/Transfer Fcn (with initial outputs)  N=[T2 1]  D=[T3 1]  Y0=P0  U0=P0
  Transfer Fcn (with initial outputs)2 : simulink_extras/Additional Linear/Transfer Fcn (with initial outputs)  N=[1]  D=[T1 1]  Y0=P0  U0=P0
  Pm : Outport
  wires:
  Transfer Fcn (with initial outputs)1/1 -> Saturation1/1
  Saturation/1 -> Transfer Fcn (with initial outputs)1/1
  Transfer Fcn (with initial outputs)2/1 -> Saturation/1
  RefL/1 -> Transfer Fcn (with initial outputs)2/1
  Saturation1/1 -> Pm/1

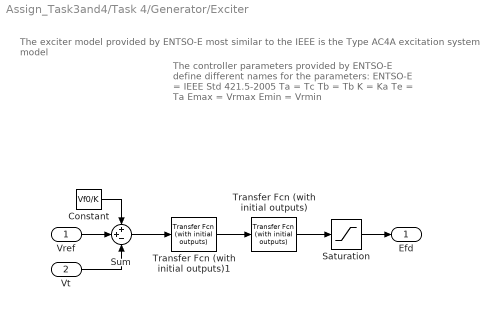
== system Assign_Task3and4/Task 4/Generator/Exciter ==
  note: The controller parameters provided by ENTSO-E
      | define different names for the parameters:
      |
      | ENTSO-E = IEEE Std 421.5-2005
      | Ta = Tc
      | Tb = Tb
      | K = Ka
      | Te = Ta
      | Emax = Vrmax
      | Emin = Vrmin
  note: The exciter model provided by ENTSO-E most similar to the IEEE is the Type AC4A excitation system model
  Vref : Inport
  Vt : Inport  Port=2
  Constant : Constant  Value=Vf0/K
  Saturation : Saturate  UpperLimit=Emax  LowerLimit=Emin
  Sum : Sum  Inputs=++-
  Transfer Fcn (with initial outputs) : simulink_extras/Additional Linear/Transfer Fcn (with initial outputs)  N=[K]  D=[Te 1]  Y0=Vf0  U0=Vf0/K
  Transfer Fcn (with initial outputs)1 : simulink_extras/Additional Linear/Transfer Fcn (with initial outputs)  N=[Ta 1]  D=[Tb 1]  Y0=Vf0/K  U0=Vf0/K
  Efd : Outport
  wires:
  Saturation/1 -> Efd/1
  Transfer Fcn (with initial outputs)1/1 -> Transfer Fcn (with initial outputs)/1
  Sum/1 -> Transfer Fcn (with initial outputs)1/1
  Transfer Fcn (with initial outputs)/1 -> Saturation/1
  Vt/1 -> Sum/3
  Vref/1 -> Sum/2
  Constant/1 -> Sum/1

== system Assign_Task3and4/Task 4/Generator/Turbine without governor ==
  note: mechanical power
  RefL : Inport
  Saturation : Saturate  UpperLimit=Vmax  LowerLimit=Vmin
  Saturation1 : Saturate  UpperLimit=1
  Transfer Fcn (with initial outputs)1 : simulink_extras/Additional Linear/Transfer Fcn (with initial outputs)  N=[T2 1]  D=[T3 1]  Y0=P0  U0=P0
  Transfer Fcn (with initial outputs)2 : simulink_extras/Additional Linear/Transfer Fcn (with initial outputs)  N=[1]  D=[T1 1]  Y0=P0  U0=P0
  Pm : Outport
  wires:
  Transfer Fcn (with initial outputs)1/1 -> Saturation1/1
  Saturation/1 -> Transfer Fcn (with initial outputs)1/1
  Transfer Fcn (with initial outputs)2/1 -> Saturation/1
  RefL/1 -> Transfer Fcn (with initial outputs)2/1
  Saturation1/1 -> Pm/1
